simulink library "cvt_powertrain_lib"  (R2026a)
settings: Solver=VariableStepAuto
undefined symbols (not defined in the file or in its folder): fluids, HMPST
libraries: fl_lib x90, nesl_utility x31, cvt_components_lib x27, sdl_lib x24, SimscapeFluids_lib x11, simulink_extras x6, $bdroot x4, ee_lib x2, batteryecm_lib x1, simulink x1, engine_mgmt_lib x1, slpidlib x1
(part 3 of 4)

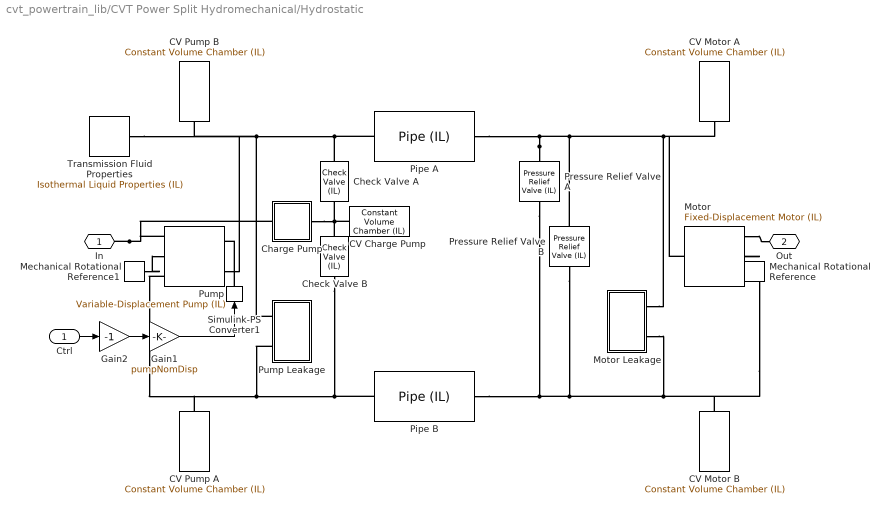
== system cvt_powertrain_lib/CVT Power Split Hydromechanical/Hydrostatic ==
  Ctrl : Inport
  CV Charge Pump : fl_lib/Isothermal Liquid/Elements/Constant Volume Chamber (IL)  volume=1e-4 m^3  p_I_specify=off  p_I_priority=High  p_I=0.101325 MPa  p_I_nominal_specify=off  p_I_nominal_value=1  p_I_nominal_unit=MPa
  CV Motor A : fl_lib/Isothermal Liquid/Elements/Constant Volume Chamber (IL)  volume=1e-4 m^3  p_I_specify=off  p_I_priority=High  p_I=0.101325 MPa  p_I_nominal_specify=off  p_I_nominal_value=1  p_I_nominal_unit=MPa
  CV Motor B : fl_lib/Isothermal Liquid/Elements/Constant Volume Chamber (IL)  volume=1e-4 m^3  p_I_specify=off  p_I_priority=High  p_I=0.101325 MPa  p_I_nominal_specify=off  p_I_nominal_value=1  p_I_nominal_unit=MPa
  CV Pump A : fl_lib/Isothermal Liquid/Elements/Constant Volume Chamber (IL)  volume=1e-4 m^3  p_I_specify=off  p_I_priority=High  p_I=0.101325 MPa  p_I_nominal_specify=off  p_I_nominal_value=1  p_I_nominal_unit=MPa
  CV Pump B : fl_lib/Isothermal Liquid/Elements/Constant Volume Chamber (IL)  volume=1e-4 m^3  p_I_specify=off  p_I_priority=High  p_I=0.101325 MPa  p_I_nominal_specify=off  p_I_nominal_value=1  p_I_nominal_unit=MPa
  Charge Pump : Subsystem  Tag=PublishSubsystem  mask{chgPumpNomDisp=chgPumpNomDisp, chgPumpNomSpd=chgPumpNomSpd, chgPumpNomPressGain=chgPumpNomPressGain, chgPumpNomVolEff=chgPumpNomVolEff, chgPumpNomMechEff=chgPumpNomMechEff, chgPumpChkvPdiff=chgPumpChkvPdiff, chgPumpChkvPrange=chgPumpChkvPrange, chgPumpChkvAmax=chgPumpChkvAmax, chgPumpChkvAleak=chgPumpChkvAleak}
      mask prompts: chgPumpNomDisp "Displacement (cm^3/rev)"; chgPumpNomSpd "Nominal Angular Velocity (rpm)"; chgPumpNomPressGain "Nominal pressure gain (MPa)"; chgPumpNomVolEff "Nominal Volumetric Efficiency (0-1)"; chgPumpNomMechEff "Nominal Mechanical Efficiency (0-1)"; chgPumpChkvPdiff "Set pressure differential (MPa)"; chgPumpChkvPrange "Pressure regulation range (MPa)"; chgPumpChkvAmax "Maximum opening area (m^2)"; chgPumpChkvAleak "Leakage area (m^2)"
      mask TypeOptions chgPumpNomDisp: Pump/displacement
      mask TypeOptions chgPumpNomSpd: Pump/omega_nominal
      mask TypeOptions chgPumpNomPressGain: Pump/p_nominal
      mask TypeOptions chgPumpNomVolEff: Pump/vol_eff_nominal
      mask TypeOptions chgPumpNomMechEff: Pump/mech_eff_nominal
      mask TypeOptions chgPumpChkvPdiff:
      | Pressure
      | Relief
      | Valve/p_set_differential
      mask TypeOptions chgPumpChkvPrange:
      | Pressure
      | Relief
      | Valve/p_range
      mask TypeOptions chgPumpChkvAmax:
      | Pressure
      | Relief
      | Valve/area_max
      mask TypeOptions chgPumpChkvAleak:
      | Pressure
      | Relief
      | Valve/area_leak
      mask DialogControl grp_chg_pump Prompt: Pump
      mask DialogControl grp_chg_pump_prv Prompt: Pressure Relief Valve
      mask Display:
      | % Circle
      | color('green')
      | plot(2*cos(linspace(0, 2*pi, 100)), 2*sin(linspace(0, 2*pi, 100)))
      | % Triangle
      | patch([1 0.4 0.4]*2, [0,-0.4,0.4]*2,[45 48 173]/255)
      | % Boundary
      | color('white')
      | plot(-2, -2)
      | plot(2, 2)
  Check Valve A : SimscapeFluids_lib/Isothermal Liquid/Valves & Orifices/Directional Control Valves/Check Valve (IL)  opening_spec=2*(fluids.isothermal_liquid.valves_orifices.enum.PressureOpeningSpec.Linear)-1  pressure_control_spec=fluids.isothermal_liquid.valves_orifices.enum.pressure_control_spec.dp  p_crack_differential=p_crack_differential MPa  p_crack_gauge=0.1 MPa  press_max_differential=press_max_differential MPa  press_max_gauge=0.2 MPa  area_max=chkv_area_max m^2  area_leak=chkv_area_leak m^2  p_diff_TLU=[0.01 : 0.01 : 0.1] MPa  valve_area_TLU=[1e-10, 1e-05, 2e-05, 3e-05, 4e-05, 5e-05, 6e-05, 7.5e-05, 8.5e-05, .0001] m^2  vol_flow_TLU=[.000358, .045, .11, .191, .284, .39, .505, .63, .764, .905] .* 1e-3 m^3/s  area=inf m^2  Cd=0.64  Re_c=150  smoothing_factor=0.01  pressure_recovery=simscape.enum.onoff.off  opening_dynamics=simscape.enum.onoff.off  tau=0.1 s
  Check Valve B : SimscapeFluids_lib/Isothermal Liquid/Valves & Orifices/Directional Control Valves/Check Valve (IL)  opening_spec=2*(fluids.isothermal_liquid.valves_orifices.enum.PressureOpeningSpec.Linear)-1  pressure_control_spec=fluids.isothermal_liquid.valves_orifices.enum.pressure_control_spec.dp  p_crack_differential=p_crack_differential MPa  p_crack_gauge=0.1 MPa  press_max_differential=press_max_differential MPa  press_max_gauge=0.2 MPa  area_max=chkv_area_max m^2  area_leak=chkv_area_leak m^2  p_diff_TLU=[0.01 : 0.01 : 0.1] MPa  valve_area_TLU=[1e-10, 1e-05, 2e-05, 3e-05, 4e-05, 5e-05, 6e-05, 7.5e-05, 8.5e-05, .0001] m^2  vol_flow_TLU=[.000358, .045, .11, .191, .284, .39, .505, .63, .764, .905] .* 1e-3 m^3/s  area=inf m^2  Cd=0.64  Re_c=150  smoothing_factor=0.01  pressure_recovery=simscape.enum.onoff.off  opening_dynamics=simscape.enum.onoff.off  tau=0.1 s
  Gain1 : Gain  Gain=pumpNomDisp
  Gain2 : Gain  Gain=-1
  Mechanical Rotational Reference : fl_lib/Mechanical/Rotational Elements/Mechanical Rotational Reference
  Mechanical Rotational Reference1 : fl_lib/Mechanical/Rotational Elements/Mechanical Rotational Reference
  Motor : SimscapeFluids_lib/Isothermal Liquid/Pumps & Motors/Fixed-Displacement Motor (IL)  leakage_friction_spec=fluids.isothermal_liquid.pumps_motors.enum.MotorLossSpec.Analytical  displacement=motorNomDisp cm^3/rev  omega_nominal=motorNomSpd rpm  p_nominal=motorNomPressDrop MPa  vol_eff_nominal=motorNomVolEff  mech_eff_nominal=motorNomMechEff  no_load_torque=0 N*m  p_diff_eff_TLU=[.1, 1, 2] MPa  omega_eff_TLU=[25, 50, 100, 200, 300, 400] rad/s  vol_eff_TLU=[.816, .908, .954, .977, .981, .984; .325, .663, .831, .916, .925, .946; .137, .568, .78, .892, .893, .91]  mech_eff_TLU=[.996, .996, .996, .996, .996, .996; .988, .989, .989, .989, .989, .99; .981, .981, .982, .982, .983, .984]  p_diff_loss_TLU=[.1, 1, 2] MPa  omega_loss_TLU=[25, 50, 100, 200, 300, 400] rad/s  vol_loss_TLU=[.023, .023, .023, .023, .0285, .032; .0844, .0842, .0845, .084, .1125, .108; .1079, .108, .11, .108, .1605, .18] * 1e-3 m^3/s  mech_loss_TLU=[.002, .002, .002, .002, .002, .002; .0607, .0556, .0556, .0556, .0556, .0505; .1937, .1937, .1833, .1833, .1729, .1626] N*m  q_shaft_TLU=[.125, .25, .5, 1, 1.5, 2] * 1e-3 m^3/s  p_diff_shaft_TLU=[.1, 1, 2] MPa  torque_shaft_TLU=[.47, 4.72, 9.35; .47, 4.7, 9.36; .47, 4.7, 9.4; .47, 4.7, 9.41; .47, 4.7, 9.46; .47, 4.68, 9.5] N*m  omega_shaft_TLU=[205, 80, 35; 455, 330, 285; 955, 831, 780; 1950, 1830, 1780; 2940, 2775, 2680; 3940, 3780, 3640] rpm  vol_eff_min=1e-3  vol_eff_max=1  mech_eff_min=1e-3  mech_eff_max=1  pressure_threshold=1e-3 MPa  omega_threshold=10 rad/s  supplied_range_check=simscape.enum.assert.action.none  motor_mode_check=simscape.enum.assert.action.none  pressure_check=simscape.enum.assert.action.none  p_min_valid=0.101325 MPa
  Motor Leakage : Subsystem  Tag=PublishSubsystem
  "Pipe A " : fl_lib/Isothermal Liquid/Elements/Pipe (IL)  length=pipeLen m  area=pipeAreaGeo m^2  Dh=pipeAreaHydr m  length_add=4 m  roughness=15e-6 m  Re_lam=2000  Re_tur=4000  shape_factor=64  dynamic_compressibility=simscape.enum.onoff.on  inertia=simscape.enum.onoff.off  p0=0.101325 MPa  mdot0=0 kg/s
  Pipe B : fl_lib/Isothermal Liquid/Elements/Pipe (IL)  length=pipeLen m  area=pipeAreaGeo m^2  Dh=pipeAreaHydr m  length_add=4 m  roughness=15e-6 m  Re_lam=2000  Re_tur=4000  shape_factor=64  dynamic_compressibility=simscape.enum.onoff.on  inertia=simscape.enum.onoff.off  p0=0.101325 MPa  mdot0=0 kg/s
  Pressure Relief Valve A : SimscapeFluids_lib/Isothermal Liquid/Valves & Orifices/Pressure Control Valves/Pressure Relief Valve (IL)  set_pressure_spec=foundation.enum.constant_controlled.constant  opening_spec=fluids.isothermal_liquid.valves_orifices.enum.opening_spec.linear  pressure_spec=fluids.isothermal_liquid.valves_orifices.enum.pressure_control_spec.dp  p_set_gauge=0.1 MPa  p_set_differential=p_set_differential MPa  p_range=p_range MPa  area_max=prv_area_max m^2  area_leak=prv_area_leak m^2  p_diff_TLU=[0.2 : 0.2 : 1.2] MPa  p_gauge_TLU=[0.2 : 0.2 : 1.2] MPa  valve_area_TLU=[1e-10, 2e-06, 4e-06, 6e-06, 8e-06, 1e-05] m^2  vol_flow_TLU=[1e-09, 3.6e-05, 8.9e-05, .00015, .00023, .00031] m^3/s  area=inf m^2  Cd=0.64  Re_c=150  smoothing_factor=0.01  pressure_recovery=simscape.enum.onoff.off  opening_dynamics=simscape.enum.onoff.off  tau=0.1 s
  Pressure Relief Valve B : SimscapeFluids_lib/Isothermal Liquid/Valves & Orifices/Pressure Control Valves/Pressure Relief Valve (IL)  set_pressure_spec=foundation.enum.constant_controlled.constant  opening_spec=fluids.isothermal_liquid.valves_orifices.enum.opening_spec.linear  pressure_spec=fluids.isothermal_liquid.valves_orifices.enum.pressure_control_spec.dp  p_set_gauge=0.1 MPa  p_set_differential=p_set_differential MPa  p_range=p_range MPa  area_max=prv_area_max m^2  area_leak=prv_area_leak m^2  p_diff_TLU=[0.2 : 0.2 : 1.2] MPa  p_gauge_TLU=[0.2 : 0.2 : 1.2] MPa  valve_area_TLU=[1e-10, 2e-06, 4e-06, 6e-06, 8e-06, 1e-05] m^2  vol_flow_TLU=[1e-09, 3.6e-05, 8.9e-05, .00015, .00023, .00031] m^3/s  area=inf m^2  Cd=0.64  Re_c=150  smoothing_factor=0.01  pressure_recovery=simscape.enum.onoff.off  opening_dynamics=simscape.enum.onoff.off  tau=0.1 s
  Pump : SimscapeFluids_lib/Isothermal Liquid/Pumps & Motors/Variable-Displacement Pump (IL)  leakage_friction_spec=fluids.isothermal_liquid.pumps_motors.enum.pump_motor_loss_spec.analytical  displacement_nominal=pumpNomDisp cm^3/rev  omega_nominal=pumpNomSpd rpm  p_nominal=pumpNomPressGain MPa  vol_eff_nominal=pumpNomVolEff  mech_eff_nominal=pumpNomMechEff  no_load_torque=0 N*m  p_diff_eff_TLU=[.1, 1, 2] MPa  omega_eff_TLU=[25, 50, 100, 200, 300, 400] rad/s  displacement_eff_TLU=[-30, -19, 19, 30] cm^3/rev  vol_eff_TLU=repmat([.816, .908, .954, .977, .981, .984; .325, .663, .831, .916, .925, .946; .137, .568, .78, .892, .893, .91], 1, 1, 4)  mech_eff_TLU=repmat([.996, .996, .996, .996, .996, .996; .988, .989, .989, .989, .989, .99; .981, .981, .982, .982, .983, .984], 1, 1, 4)  p_diff_loss_TLU=[.1, 1, 2] MPa  omega_loss_TLU=[25, 50, 100, 200, 300, 400] rad/s  displacement_loss_TLU=[-30, -19, 19, 30] cm^3/rev  vol_loss_TLU=repmat([.023, .023, .023, .023, .0285, .032; .0844, .0842, .0845, .084, .1125, .108; .1079, .108, .11, .108, .1605, .18] * 1e-3, 1, 1, 4) m^3/s  mech_loss_TLU=repmat([.002, .002, .002, .002, .002, .002; .0607, .0556, .0556, .0556, .0556, .0505; .1937, .1937, .1833, .1833, .1729, .1626], 1, 1, 4) N*m  vol_eff_min=1e-3  vol_eff_max=1  mech_eff_min=1e-3  mech_eff_max=1  pressure_threshold=1e-3 MPa  omega_threshold=10 rad/s  displacement_threshold=0.1 cm^3/rev  supplied_range_check=simscape.enum.assert.action.none  pump_mode_check=simscape.enum.assert.action.none  pressure_check=simscape.enum.assert.action.none  p_min_valid=0.101325 MPa
  Pump Leakage : Subsystem  Tag=PublishSubsystem
  Simulink-PS Converter1 : nesl_utility/Simulink-PS Converter  PhysicalDomain=network_engine_domain  SubClassName=ps_input  LeftPortType=input  RightPortType=output  PseudoPeriodic=off  Frequencies=[]  NoiseDistribution=none  NoiseParameters=[]  Unit=cm^3/rev  AffineConversion=off  FilteringAndDerivatives=provide  SimscapeFilterOrder=1  InputFilterTimeConstant=0.001  UdotUserProvided=0
  Transmission Fluid Properties : fl_lib/Isothermal Liquid/Utilities/Isothermal Liquid Properties (IL)  rho_L_atm=850 kg/m^3  bulk_modulus_model=foundation.enum.bulk_modulus_model.const  beta_gain=6  beta_L_atm=1.4 GPa  nu_atm=18.8 cSt  p_atm=0.101325 MPa  p_min=0.1 Pa  properties_range_check=simscape.enum.assert.action.error  air_fraction=0.005  polytropic_index=1.0  rho_g_atm=1.225 kg/m^3  air_dissolution_model=simscape.enum.onoff.off  p_crit=3 MPa
  In : PMIOPort  Side=Left
  Out : PMIOPort  Port=2  Side=Right
  wires:
  Ctrl/1 -> Gain2/1
  Gain1/1 -> Simulink-PS Converter1/1
  Gain2/1 -> Gain1/1
  connections:
  In/RConn1 -- Charge Pump/LConn1 -- Pump/RConn1
  Motor/RConn1 -- Out/RConn1
  Mechanical Rotational Reference1/LConn1 -- Pump/RConn2
  Pressure Relief Valve A/LConn1 -- Pressure Relief Valve B/RConn1 -- Motor Leakage/LConn1 -- CV Motor A/LConn1 -- Motor/LConn1 -- "Pipe A "/RConn1
  Motor/RConn2 -- Mechanical Rotational Reference/LConn1
  Check Valve B/LConn1 -- Check Valve A/LConn1 -- Charge Pump/RConn1 -- CV Charge Pump/LConn1
  Check Valve A/RConn1 -- Pump Leakage/LConn1 -- Transmission Fluid Properties/RConn1 -- CV Pump B/LConn1 -- Pump/LConn2 -- "Pipe A "/LConn1
  Check Valve B/RConn1 -- Pump Leakage/LConn2 -- CV Pump A/LConn1 -- Pump/RConn3 -- Pipe B/LConn1
  Pressure Relief Valve A/RConn1 -- Pressure Relief Valve B/LConn1 -- Motor Leakage/LConn2 -- CV Motor B/LConn1 -- Motor/RConn3 -- Pipe B/RConn1
  Simulink-PS Converter1/RConn1 -- Pump/LConn1

== system cvt_powertrain_lib/CVT Power Split Hydromechanical/Sensor P1s ==
  MRRef : fl_lib/Mechanical/Rotational Elements/Mechanical Rotational Reference
  Motion Sensor : fl_lib/Mechanical/Mechanical Sensors/Ideal Rotational Motion Sensor  reference=foundation.enum.MeasurementReference.difference  acceleration_port=false  velocity_port=true  position_port=false  wrap_angle=false  offset=0 rad
  PS-Simulink Converter : nesl_utility/PS-Simulink Converter  PhysicalDomain=network_engine_domain  SubClassName=ps_output  LeftPortType=input  RightPortType=output  PseudoPeriodic=off  Frequencies=[]  VectorFormat=inherit  Unit=rpm  AffineConversion=off
  R : PMIOPort  Side=Left
  w : Outport
  wires:
  PS-Simulink Converter/1 -> w/1
  connections:
  R/RConn1 -- Motion Sensor/LConn1
  MRRef/LConn1 -- Motion Sensor/RConn1
  PS-Simulink Converter/LConn1 -- Motion Sensor/RConn2

== system cvt_powertrain_lib/CVT Power Split Hydromechanical/Sensor wG2 ==
  MRRef : fl_lib/Mechanical/Rotational Elements/Mechanical Rotational Reference
  Motion Sensor : fl_lib/Mechanical/Mechanical Sensors/Ideal Rotational Motion Sensor  reference=foundation.enum.MeasurementReference.difference  acceleration_port=false  velocity_port=true  position_port=false  wrap_angle=false  offset=0 rad
  PS-Simulink Converter : nesl_utility/PS-Simulink Converter  PhysicalDomain=network_engine_domain  SubClassName=ps_output  LeftPortType=input  RightPortType=output  PseudoPeriodic=off  Frequencies=[]  VectorFormat=inherit  Unit=rpm  AffineConversion=off
  R : PMIOPort  Side=Left
  w : Outport
  wires:
  PS-Simulink Converter/1 -> w/1
  connections:
  R/RConn1 -- Motion Sensor/LConn1
  MRRef/LConn1 -- Motion Sensor/RConn1
  PS-Simulink Converter/LConn1 -- Motion Sensor/RConn2

== system cvt_powertrain_lib/CVT Power Split Hydromechanical/Sensor wG3 ==
  MRRef : fl_lib/Mechanical/Rotational Elements/Mechanical Rotational Reference
  Motion Sensor : fl_lib/Mechanical/Mechanical Sensors/Ideal Rotational Motion Sensor  reference=foundation.enum.MeasurementReference.difference  acceleration_port=false  velocity_port=true  position_port=false  wrap_angle=false  offset=0 rad
  PS-Simulink Converter : nesl_utility/PS-Simulink Converter  PhysicalDomain=network_engine_domain  SubClassName=ps_output  LeftPortType=input  RightPortType=output  PseudoPeriodic=off  Frequencies=[]  VectorFormat=inherit  Unit=rpm  AffineConversion=off
  R : PMIOPort  Side=Left
  w : Outport
  wires:
  PS-Simulink Converter/1 -> w/1
  connections:
  PS-Simulink Converter/LConn1 -- Motion Sensor/RConn2
  MRRef/LConn1 -- Motion Sensor/RConn1
  R/RConn1 -- Motion Sensor/LConn1

== system cvt_powertrain_lib/CVT Power Split Hydromechanical/Sensor wG4 ==
  MRRef : fl_lib/Mechanical/Rotational Elements/Mechanical Rotational Reference
  Motion Sensor : fl_lib/Mechanical/Mechanical Sensors/Ideal Rotational Motion Sensor  reference=foundation.enum.MeasurementReference.difference  acceleration_port=false  velocity_port=true  position_port=false  wrap_angle=false  offset=0 rad
  PS-Simulink Converter : nesl_utility/PS-Simulink Converter  PhysicalDomain=network_engine_domain  SubClassName=ps_output  LeftPortType=input  RightPortType=output  PseudoPeriodic=off  Frequencies=[]  VectorFormat=inherit  Unit=rpm  AffineConversion=off
  R : PMIOPort  Side=Left
  w : Outport
  wires:
  PS-Simulink Converter/1 -> w/1
  connections:
  PS-Simulink Converter/LConn1 -- Motion Sensor/RConn2
  MRRef/LConn1 -- Motion Sensor/RConn1
  R/RConn1 -- Motion Sensor/LConn1

== system cvt_powertrain_lib/CVT Power Split Hydromechanical/Sensor wIn ==
  MRRef : fl_lib/Mechanical/Rotational Elements/Mechanical Rotational Reference
  Motion Sensor : fl_lib/Mechanical/Mechanical Sensors/Ideal Rotational Motion Sensor  reference=foundation.enum.MeasurementReference.difference  acceleration_port=false  velocity_port=true  position_port=false  wrap_angle=false  offset=0 rad
  PS-Simulink Converter : nesl_utility/PS-Simulink Converter  PhysicalDomain=network_engine_domain  SubClassName=ps_output  LeftPortType=input  RightPortType=output  PseudoPeriodic=off  Frequencies=[]  VectorFormat=inherit  Unit=rpm  AffineConversion=off
  R : PMIOPort  Side=Left
  w : Outport
  wires:
  PS-Simulink Converter/1 -> w/1
  connections:
  PS-Simulink Converter/LConn1 -- Motion Sensor/RConn2
  MRRef/LConn1 -- Motion Sensor/RConn1
  R/RConn1 -- Motion Sensor/LConn1

== system cvt_powertrain_lib/CVT Power Split Hydromechanical/Sensor wOut ==
  MRRef : fl_lib/Mechanical/Rotational Elements/Mechanical Rotational Reference
  Motion Sensor : fl_lib/Mechanical/Mechanical Sensors/Ideal Rotational Motion Sensor  reference=foundation.enum.MeasurementReference.difference  acceleration_port=false  velocity_port=true  position_port=false  wrap_angle=false  offset=0 rad
  PS-Simulink Converter : nesl_utility/PS-Simulink Converter  PhysicalDomain=network_engine_domain  SubClassName=ps_output  LeftPortType=input  RightPortType=output  PseudoPeriodic=off  Frequencies=[]  VectorFormat=inherit  Unit=rpm  AffineConversion=off
  R : PMIOPort  Side=Left
  w : Outport
  wires:
  PS-Simulink Converter/1 -> w/1
  connections:
  R/RConn1 -- Motion Sensor/LConn1
  MRRef/LConn1 -- Motion Sensor/RConn1
  PS-Simulink Converter/LConn1 -- Motion Sensor/RConn2

== system cvt_powertrain_lib/CVT Power Split Hydromechanical/Sensor wP1c ==
  MRRef : fl_lib/Mechanical/Rotational Elements/Mechanical Rotational Reference
  Motion Sensor : fl_lib/Mechanical/Mechanical Sensors/Ideal Rotational Motion Sensor  reference=foundation.enum.MeasurementReference.difference  acceleration_port=false  velocity_port=true  position_port=false  wrap_angle=false  offset=0 rad
  PS-Simulink Converter : nesl_utility/PS-Simulink Converter  PhysicalDomain=network_engine_domain  SubClassName=ps_output  LeftPortType=input  RightPortType=output  PseudoPeriodic=off  Frequencies=[]  VectorFormat=inherit  Unit=rpm  AffineConversion=off
  R : PMIOPort  Side=Left
  w : Outport
  wires:
  PS-Simulink Converter/1 -> w/1
  connections:
  R/RConn1 -- Motion Sensor/LConn1
  MRRef/LConn1 -- Motion Sensor/RConn1
  PS-Simulink Converter/LConn1 -- Motion Sensor/RConn2

== system cvt_powertrain_lib/CVT Power Split Hydromechanical/Sensor wP2s ==
  MRRef : fl_lib/Mechanical/Rotational Elements/Mechanical Rotational Reference
  Motion Sensor : fl_lib/Mechanical/Mechanical Sensors/Ideal Rotational Motion Sensor  reference=foundation.enum.MeasurementReference.difference  acceleration_port=false  velocity_port=true  position_port=false  wrap_angle=false  offset=0 rad
  PS-Simulink Converter : nesl_utility/PS-Simulink Converter  PhysicalDomain=network_engine_domain  SubClassName=ps_output  LeftPortType=input  RightPortType=output  PseudoPeriodic=off  Frequencies=[]  VectorFormat=inherit  Unit=rpm  AffineConversion=off
  R : PMIOPort  Side=Left
  w : Outport
  wires:
  PS-Simulink Converter/1 -> w/1
  connections:
  PS-Simulink Converter/LConn1 -- Motion Sensor/RConn2
  MRRef/LConn1 -- Motion Sensor/RConn1
  R/RConn1 -- Motion Sensor/LConn1

== system cvt_powertrain_lib/CVT Power Split Hydromechanical/Sensor wP3r ==
  MRRef : fl_lib/Mechanical/Rotational Elements/Mechanical Rotational Reference
  Motion Sensor : fl_lib/Mechanical/Mechanical Sensors/Ideal Rotational Motion Sensor  reference=foundation.enum.MeasurementReference.difference  acceleration_port=false  velocity_port=true  position_port=false  wrap_angle=false  offset=0 rad
  PS-Simulink Converter : nesl_utility/PS-Simulink Converter  PhysicalDomain=network_engine_domain  SubClassName=ps_output  LeftPortType=input  RightPortType=output  PseudoPeriodic=off  Frequencies=[]  VectorFormat=inherit  Unit=rpm  AffineConversion=off
  R : PMIOPort  Side=Left
  w : Outport
  wires:
  PS-Simulink Converter/1 -> w/1
  connections:
  PS-Simulink Converter/LConn1 -- Motion Sensor/RConn2
  MRRef/LConn1 -- Motion Sensor/RConn1
  R/RConn1 -- Motion Sensor/LConn1

== system cvt_powertrain_lib/CVT Power Split Hydromechanical/Sensor wP4c ==
  MRRef : fl_lib/Mechanical/Rotational Elements/Mechanical Rotational Reference
  Motion Sensor : fl_lib/Mechanical/Mechanical Sensors/Ideal Rotational Motion Sensor  reference=foundation.enum.MeasurementReference.difference  acceleration_port=false  velocity_port=true  position_port=false  wrap_angle=false  offset=0 rad
  PS-Simulink Converter : nesl_utility/PS-Simulink Converter  PhysicalDomain=network_engine_domain  SubClassName=ps_output  LeftPortType=input  RightPortType=output  PseudoPeriodic=off  Frequencies=[]  VectorFormat=inherit  Unit=rpm  AffineConversion=off
  R : PMIOPort  Side=Left
  w : Outport
  wires:
  PS-Simulink Converter/1 -> w/1
  connections:
  PS-Simulink Converter/LConn1 -- Motion Sensor/RConn2
  MRRef/LConn1 -- Motion Sensor/RConn1
  R/RConn1 -- Motion Sensor/LConn1

== system cvt_powertrain_lib/CVT Power Split Hydromechanical/Sensor wP4r ==
  MRRef : fl_lib/Mechanical/Rotational Elements/Mechanical Rotational Reference
  Motion Sensor : fl_lib/Mechanical/Mechanical Sensors/Ideal Rotational Motion Sensor  reference=foundation.enum.MeasurementReference.difference  acceleration_port=false  velocity_port=true  position_port=false  wrap_angle=false  offset=0 rad
  PS-Simulink Converter : nesl_utility/PS-Simulink Converter  PhysicalDomain=network_engine_domain  SubClassName=ps_output  LeftPortType=input  RightPortType=output  PseudoPeriodic=off  Frequencies=[]  VectorFormat=inherit  Unit=rpm  AffineConversion=off
  R : PMIOPort  Side=Left
  w : Outport
  wires:
  PS-Simulink Converter/1 -> w/1
  connections:
  R/RConn1 -- Motion Sensor/LConn1
  MRRef/LConn1 -- Motion Sensor/RConn1
  PS-Simulink Converter/LConn1 -- Motion Sensor/RConn2

== system cvt_powertrain_lib/CVT Power Split Hydromechanical/Sensor wP4s ==
  MRRef : fl_lib/Mechanical/Rotational Elements/Mechanical Rotational Reference
  Motion Sensor : fl_lib/Mechanical/Mechanical Sensors/Ideal Rotational Motion Sensor  reference=foundation.enum.MeasurementReference.difference  acceleration_port=false  velocity_port=true  position_port=false  wrap_angle=false  offset=0 rad
  PS-Simulink Converter : nesl_utility/PS-Simulink Converter  PhysicalDomain=network_engine_domain  SubClassName=ps_output  LeftPortType=input  RightPortType=output  PseudoPeriodic=off  Frequencies=[]  VectorFormat=inherit  Unit=rpm  AffineConversion=off
  R : PMIOPort  Side=Left
  w : Outport
  wires:
  PS-Simulink Converter/1 -> w/1
  connections:
  PS-Simulink Converter/LConn1 -- Motion Sensor/RConn2
  MRRef/LConn1 -- Motion Sensor/RConn1
  R/RConn1 -- Motion Sensor/LConn1

== system cvt_powertrain_lib/Controller/CVT Ratio Ctrl ==
  Ratio (-) : Inport
  CmdVehSpdDir : Inport  Port=2
  HRBCtrl (-) : Inport  Port=3
  MBCtrl (-) : Inport  Port=4
  Bus Creator : BusCreator  Inputs=12
  Clutch Truth Table : Stateflow chart  TreatAsAtomicUnit=on
  Filter : StateSpace  A=-200  C=200  D=0  InitialCondition=HMPST.Ctrl.Swash.XY_A(1,1)/200
  Range Calculation : Subsystem  mask{XY_I=HMPST.Ctrl.Swash.XY_I}
      mask prompts: XY_I "Range Separation Points"
  Saturation : Saturate  UpperLimit=HMPST.DesignReq.MaxCVTOutputSpeed/HMPST.Eng.wTarget  LowerLimit=0  ZeroCross=off
  Swash Ctrl : Lookup_n-D  NumberOfTableDimensions=1  BreakpointsForDimension1=HMPST.Ctrl.Swash.XY_A(:,2)  BeginIndexSearchUsingPreviousIndexResult=on  Table=HMPST.Ctrl.Swash.XY_A(:,1)  InternalRulePriority=Speed  RndMeth=Simplest
  Transfer Fcn : TransferFcn  Denominator=[0.1 1]
  CVT Ctrl : Outport
  wires:
  Ratio (-)/1 -> [ratio], Transfer Fcn/1
  Clutch Truth Table/1(K1Actv) -> Bus Creator/1  "K1"
  Clutch Truth Table/2(K2Actv) -> Bus Creator/2  "K2"
  Clutch Truth Table/3(K3Actv) -> Bus Creator/3  "K3"
  Clutch Truth Table/4(K4Actv) -> Bus Creator/4  "K4"
  Clutch Truth Table/5(KbActv) -> Bus Creator/5  "Kb"
  Clutch Truth Table/6(KvActv) -> Bus Creator/6  "Kv"
  Clutch Truth Table/7(KrActv) -> Bus Creator/7  "Kr"
  Bus Creator/1 -> CVT Ctrl/1  "Ctrl"
  Range Calculation/1(Range (-)) -> Clutch Truth Table/1(Range)
  Saturation/1 -> Swash Ctrl/1, Range Calculation/1(Ratio (-))
  Transfer Fcn/1 -> Saturation/1
  Filter/1 -> Bus Creator/12  "SwashCtrl"
  Swash Ctrl/1 -> Filter/1  "SwashCtrl"
  HRBCtrl (-)/1 -> Bus Creator/8  "HRBCtrl"
  MBCtrl (-)/1 -> Bus Creator/9  "MBCtrl"
  CmdVehSpdDir/1 -> Bus Creator/11, Clutch Truth Table/2(CmdVehSpdDir)  "CmdVehSpdDir"
  [ratio] -> Bus Creator/10  "ratio"

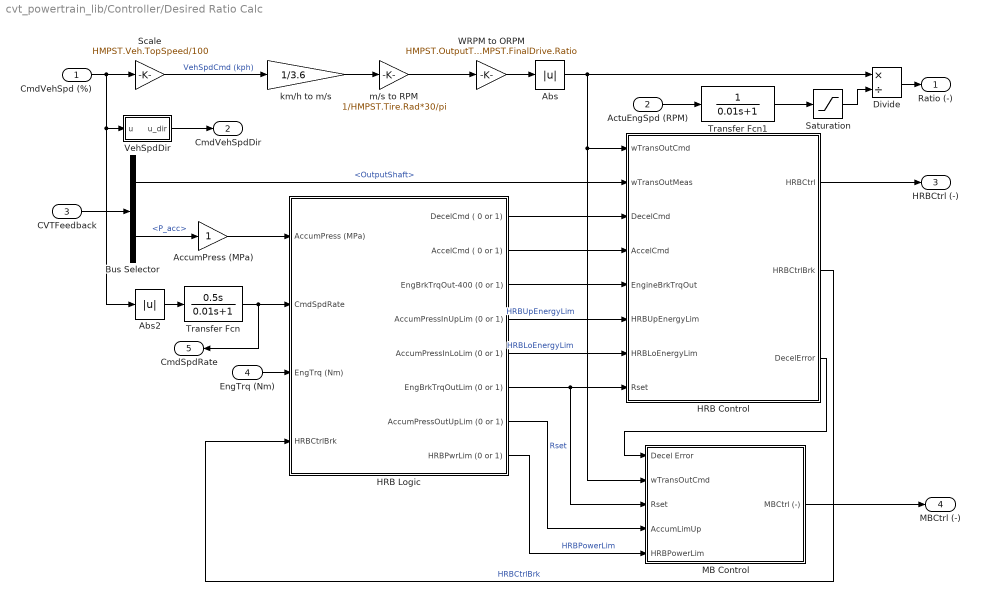
== system cvt_powertrain_lib/Controller/Desired Ratio Calc ==
  CmdVehSpd (%) : Inport  SampleTime=HMPST.Simu.TimeStep
  ActuEngSpd (RPM) : Inport  Port=2
  CVTFeedback : Inport  Port=3
  EngTrq (Nm) : Inport  Port=4
  Abs : Abs  ZeroCross=off  SaturateOnIntegerOverflow=off
  Abs2 : Abs  ZeroCross=off  SaturateOnIntegerOverflow=off
  AccumPress (MPa) : Gain
  Bus Selector : BusSelector  OutputSignals=OutputShaft,P_acc
  Divide : Product  Inputs=*/
  HRB Control : Subsystem
  HRB Logic : Subsystem
  MB Control : Subsystem
  Saturation : Saturate  UpperLimit=2500  LowerLimit=0.5
  Scale : Gain  Gain=HMPST.Veh.TopSpeed/100
  Transfer Fcn : TransferFcn  Numerator=[0.5 0]  Denominator=[0.01 1]
  Transfer Fcn1 : TransferFcn  Denominator=[0.01 1]
  VehSpdDir : Subsystem
  WRPM to ORPM : Gain  Gain=HMPST.OutputTransferGearPair.Ratio*HMPST.Differential.Ratio*HMPST.FinalDrive.Ratio
  km/h to m/s : Gain  Gain=1/3.6
  m/s to RPM : Gain  Gain=1/HMPST.Tire.Rad*30/pi
  Ratio (-) : Outport
  CmdVehSpdDir : Outport  Port=2
  HRBCtrl (-) : Outport  Port=3
  MBCtrl (-) : Outport  Port=4
  CmdSpdRate : Outport  Port=5
  wires:
  HRB Logic/8(HRBPwrLim (0 or 1)) -> MB Control/5(HRBPowerLim)  "HRBPowerLim"
  HRB Logic/7(AccumPressOutUpLim (0 or 1)) -> MB Control/4(AccumLimUp)
  HRB Control/3(DecelError) -> MB Control/1(Decel Error)
  HRB Control/1(HRBCtrl) -> HRBCtrl (-)/1
  HRB Logic/3(EngBrkTrqOut-400 (0 or 1)) -> HRB Control/5(EngineBrkTrqOut)
  HRB Logic/2(AccelCmd ( 0 or 1)) -> HRB Control/4(AccelCmd)
  HRB Logic/5(AccumPressInLoLim (0 or 1)) -> HRB Control/7(HRBLoEnergyLim)  "HRBLoEnergyLim"
  HRB Logic/4(AccumPressInUpLim (0 or 1)) -> HRB Control/6(HRBUpEnergyLim)  "HRBUpEnergyLim"
  HRB Logic/1(DecelCmd ( 0 or 1)) -> HRB Control/3(DecelCmd)
  Divide/1 -> Ratio (-)/1
  ActuEngSpd (RPM)/1 -> Transfer Fcn1/1
  m/s to RPM/1 -> WRPM to ORPM/1
  km/h to m/s/1 -> m/s to RPM/1
  WRPM to ORPM/1 -> Abs/1
  CmdVehSpd (%)/1 -> Abs2/1, VehSpdDir/1(u), Scale/1
  Saturation/1 -> Divide/2
  Transfer Fcn1/1 -> Saturation/1
  Bus Selector/1 -> HRB Control/2(wTransOutMeas)  "<OutputShaft>"
  Transfer Fcn/1 -> HRB Logic/2(CmdSpdRate), CmdSpdRate/1
  CVTFeedback/1 -> Bus Selector/1
  HRB Logic/6(EngBrkTrqOutLim (0 or 1)) -> MB Control/3(Rset), HRB Control/8(Rset)  "Rset"
  Bus Selector/2 -> AccumPress (MPa)/1  "<P_acc>"
  EngTrq (Nm)/1 -> HRB Logic/3(EngTrq (Nm))
  AccumPress (MPa)/1 -> HRB Logic/1(AccumPress (MPa))
  VehSpdDir/1(u_dir) -> CmdVehSpdDir/1
  Scale/1 -> km/h to m/s/1  "VehSpdCmd (kph)"
  Abs2/1 -> Transfer Fcn/1
  Abs/1 -> Divide/1, MB Control/2(wTransOutCmd), HRB Control/1(wTransOutCmd)
  MB Control/1(MBCtrl (-)) -> MBCtrl (-)/1
  HRB Control/2(HRBCtrlBrk) -> HRB Logic/4(HRBCtrlBrk)  "HRBCtrlBrk"

== system cvt_powertrain_lib/Driveline/Compliance FL ==
  Damper : fl_lib/Mechanical/Rotational Elements/Rotational Damper  D=HMPST.DriveshaftF.D N*m*s/rad  w_specify=off  w_priority=None  w=0 rad/s  w_nominal_specify=off  w_nominal_value=1  w_nominal_unit=rad/s  t_specify=off  t_priority=None  t=0 N*m  t_nominal_specify=off  t_nominal_value=1  t_nominal_unit=N*m
  Spring : fl_lib/Mechanical/Rotational Elements/Rotational Spring  spr_rate=HMPST.DriveshaftF.K N*m/rad  w_specify=off  w_priority=None  w=0 rad/s  w_nominal_specify=off  w_nominal_value=1  w_nominal_unit=rad/s  t_specify=off  t_priority=None  t=0 N*m  t_nominal_specify=off  t_nominal_value=1  t_nominal_unit=N*m  phi_specify=off  phi_priority=High  phi=0 rad  phi_nominal_specify=off  phi_nominal_value=1  phi_nominal_unit=rad
  R : PMIOPort  Side=Right
  C : PMIOPort  Port=2  Side=Left
  connections:
  Damper/LConn1 -- Spring/LConn1 -- R/RConn1
  Damper/RConn1 -- Spring/RConn1 -- C/RConn1

== system cvt_powertrain_lib/Driveline/Compliance FR ==
  Damper : fl_lib/Mechanical/Rotational Elements/Rotational Damper  D=HMPST.DriveshaftF.D N*m*s/rad  w_specify=off  w_priority=None  w=0 rad/s  w_nominal_specify=off  w_nominal_value=1  w_nominal_unit=rad/s  t_specify=off  t_priority=None  t=0 N*m  t_nominal_specify=off  t_nominal_value=1  t_nominal_unit=N*m
  Spring : fl_lib/Mechanical/Rotational Elements/Rotational Spring  spr_rate=HMPST.DriveshaftF.K N*m/rad  w_specify=off  w_priority=None  w=0 rad/s  w_nominal_specify=off  w_nominal_value=1  w_nominal_unit=rad/s  t_specify=off  t_priority=None  t=0 N*m  t_nominal_specify=off  t_nominal_value=1  t_nominal_unit=N*m  phi_specify=off  phi_priority=High  phi=0 rad  phi_nominal_specify=off  phi_nominal_value=1  phi_nominal_unit=rad
  R : PMIOPort  Side=Right
  C : PMIOPort  Port=2  Side=Left
  connections:
  C/RConn1 -- Damper/RConn1 -- Spring/RConn1
  R/RConn1 -- Spring/LConn1 -- Damper/LConn1

== system cvt_powertrain_lib/Driveline/Compliance RL ==
  Damper : fl_lib/Mechanical/Rotational Elements/Rotational Damper  D=HMPST.DriveshaftF.D N*m*s/rad  w_specify=off  w_priority=None  w=0 rad/s  w_nominal_specify=off  w_nominal_value=1  w_nominal_unit=rad/s  t_specify=off  t_priority=None  t=0 N*m  t_nominal_specify=off  t_nominal_value=1  t_nominal_unit=N*m
  Spring : fl_lib/Mechanical/Rotational Elements/Rotational Spring  spr_rate=HMPST.DriveshaftF.K N*m/rad  w_specify=off  w_priority=None  w=0 rad/s  w_nominal_specify=off  w_nominal_value=1  w_nominal_unit=rad/s  t_specify=off  t_priority=None  t=0 N*m  t_nominal_specify=off  t_nominal_value=1  t_nominal_unit=N*m  phi_specify=off  phi_priority=High  phi=0 rad  phi_nominal_specify=off  phi_nominal_value=1  phi_nominal_unit=rad
  R : PMIOPort  Side=Right
  C : PMIOPort  Port=2  Side=Left
  connections:
  C/RConn1 -- Damper/RConn1 -- Spring/RConn1
  R/RConn1 -- Spring/LConn1 -- Damper/LConn1

== system cvt_powertrain_lib/Driveline/Compliance RR ==
  Damper : fl_lib/Mechanical/Rotational Elements/Rotational Damper  D=HMPST.DriveshaftF.D N*m*s/rad  w_specify=off  w_priority=None  w=0 rad/s  w_nominal_specify=off  w_nominal_value=1  w_nominal_unit=rad/s  t_specify=off  t_priority=None  t=0 N*m  t_nominal_specify=off  t_nominal_value=1  t_nominal_unit=N*m
  Spring : fl_lib/Mechanical/Rotational Elements/Rotational Spring  spr_rate=HMPST.DriveshaftF.K N*m/rad  w_specify=off  w_priority=None  w=0 rad/s  w_nominal_specify=off  w_nominal_value=1  w_nominal_unit=rad/s  t_specify=off  t_priority=None  t=0 N*m  t_nominal_specify=off  t_nominal_value=1  t_nominal_unit=N*m  phi_specify=off  phi_priority=High  phi=0 rad  phi_nominal_specify=off  phi_nominal_value=1  phi_nominal_unit=rad
  R : PMIOPort  Side=Right
  C : PMIOPort  Port=2  Side=Left
  connections:
  C/RConn1 -- Damper/RConn1 -- Spring/RConn1
  R/RConn1 -- Spring/LConn1 -- Damper/LConn1

== system cvt_powertrain_lib/Engine Droop/Speed Sensor ==
  MRRef : fl_lib/Mechanical/Rotational Elements/Mechanical Rotational Reference
  Motion Sensor : fl_lib/Mechanical/Mechanical Sensors/Ideal Rotational Motion Sensor  reference=foundation.enum.MeasurementReference.difference  acceleration_port=false  velocity_port=true  position_port=false  wrap_angle=false  offset=0 rad
  Press A3 : nesl_utility/PS-Simulink Converter  PhysicalDomain=network_engine_domain  SubClassName=ps_output  LeftPortType=input  RightPortType=output  PseudoPeriodic=off  Frequencies=[]  VectorFormat=1-D array  Unit=rpm  AffineConversion=off
  Transfer Fcn : TransferFcn  Denominator=[0.1 1]
  R : PMIOPort  Side=Left
  rpm : Outport
  wires:
  Transfer Fcn/1 -> rpm/1
  Press A3/1 -> Transfer Fcn/1
  connections:
  R/RConn1 -- Motion Sensor/LConn1
  MRRef/LConn1 -- Motion Sensor/RConn1
  Motion Sensor/RConn2 -- Press A3/LConn1

== system cvt_powertrain_lib/Engine Droop/Torque Sensor ==
  PS-Simulink Converter : nesl_utility/PS-Simulink Converter  PhysicalDomain=network_engine_domain  SubClassName=ps_output  LeftPortType=input  RightPortType=output  PseudoPeriodic=off  Frequencies=[]  VectorFormat=inherit  Unit=inherit  AffineConversion=off
  Torque Sensor : fl_lib/Mechanical/Mechanical Sensors/Ideal Torque Sensor
  R : PMIOPort  Side=Left
  C : PMIOPort  Port=2  Side=Right
  m : Outport
  wires:
  PS-Simulink Converter/1 -> m/1
  connections:
  PS-Simulink Converter/LConn1 -- Torque Sensor/RConn2
  Torque Sensor/LConn1 -- R/RConn1
  C/RConn1 -- Torque Sensor/RConn1

== system cvt_powertrain_lib/Engine Generic/Speed Sensor ==
  Ideal Rotational Motion Sensor1 : fl_lib/Mechanical/Mechanical Sensors/Ideal Rotational Motion Sensor  reference=foundation.enum.MeasurementReference.difference  acceleration_port=false  velocity_port=true  position_port=false  wrap_angle=false  offset=0 rad
  Mechanical Rotational Reference1 : fl_lib/Mechanical/Rotational Elements/Mechanical Rotational Reference
  Press A3 : nesl_utility/PS-Simulink Converter  PhysicalDomain=network_engine_domain  SubClassName=ps_output  LeftPortType=input  RightPortType=output  PseudoPeriodic=off  Frequencies=[]  VectorFormat=1-D array  Unit=rpm  AffineConversion=off
  Transfer Fcn : TransferFcn  Denominator=[0.1 1]
  R : PMIOPort  Side=Left
  w (rpm) : Outport
  wires:
  Transfer Fcn/1 -> w (rpm)/1
  Press A3/1 -> Transfer Fcn/1
  connections:
  R/RConn1 -- Ideal Rotational Motion Sensor1/LConn1
  Mechanical Rotational Reference1/LConn1 -- Ideal Rotational Motion Sensor1/RConn1
  Ideal Rotational Motion Sensor1/RConn2 -- Press A3/LConn1

== system cvt_powertrain_lib/Engine Generic/Subsystem ==
  Ideal Torque Sensor : fl_lib/Mechanical/Mechanical Sensors/Ideal Torque Sensor
  PS-Simulink Converter : nesl_utility/PS-Simulink Converter  PhysicalDomain=network_engine_domain  SubClassName=ps_output  LeftPortType=input  RightPortType=output  PseudoPeriodic=off  Frequencies=[]  VectorFormat=inherit  Unit=inherit  AffineConversion=off
  R : PMIOPort  Side=Left
  C : PMIOPort  Port=2  Side=Right
  m : Outport
  wires:
  PS-Simulink Converter/1 -> m/1
  connections:
  PS-Simulink Converter/LConn1 -- Ideal Torque Sensor/RConn2
  Ideal Torque Sensor/LConn1 -- R/RConn1
  C/RConn1 -- Ideal Torque Sensor/RConn1

== system cvt_powertrain_lib/CVT Electrical/Control/Control ==
  wCmd : Inport
  wMeas : Inport  Port=2
  Integrator : Integrator
  Ki : Gain  Gain=HMPST.eCVT.Control.Ki
  Kp : Gain  Gain=HMPST.eCVT.Control.Kp
  Sum : Sum  Inputs=+-|
  Sum1 : Sum  Inputs=++|
  Transfer Fcn (with initial states) : simulink_extras/Additional Linear/Transfer Fcn (with initial states)  N=[1]  D="[HMPST.eCVT.Control.tFilt  1]"  X0=0
  Trq : Outport
  wires:
  Sum/1 -> Transfer Fcn (with initial states)/1
  Sum1/1 -> Trq/1
  Kp/1 -> Sum1/2
  Ki/1 -> Integrator/1
  Integrator/1 -> Sum1/1
  Transfer Fcn (with initial states)/1 -> Ki/1, Kp/1
  wMeas/1 -> Sum/2
  wCmd/1 -> Sum/1

== system cvt_powertrain_lib/CVT Power Split Hydromechanical/HRB/Subsystem ==
  Hydraulic Pressure Sensor : fl_lib/Isothermal Liquid/Sensors/Pressure Sensor (IL)  pressure_measure=foundation.enum.pressure_measure.difference
      settings: LibrarySourceBlock=|
      | fl_lib/Hydraulic/Hydraulic Sensors/Hydraulic Pressure
      | Sensor
  Hydraulic Reference1 : fl_lib/Isothermal Liquid/Elements/Reservoir (IL)  pressure_input=false  pressure_spec=foundation.enum.pressure_spec.atmospheric  reservoir_pressure=0.101325 MPa
      settings: LibrarySourceBlock=fl_lib/Hydraulic/Hydraulic Elements/Hydraulic Reference
  PS-Simulink Converter : nesl_utility/PS-Simulink Converter  PhysicalDomain=network_engine_domain  SubClassName=ps_output  LeftPortType=input  RightPortType=output  PseudoPeriodic=off  Frequencies=[]  VectorFormat=1-D array  Unit=MPa  AffineConversion=off
  A : PMIOPort  Side=Left
  p : Outport
  wires:
  PS-Simulink Converter/1 -> p/1
  connections:
  Hydraulic Pressure Sensor/RConn1 -- Hydraulic Reference1/LConn1
  A/RConn1 -- Hydraulic Pressure Sensor/LConn1
  Hydraulic Pressure Sensor/RConn2 -- PS-Simulink Converter/LConn1

== system cvt_powertrain_lib/CVT Power Split Hydromechanical/Hydrostatic/Charge Pump ==
  Mechanical Rotational Reference : fl_lib/Mechanical/Rotational Elements/Mechanical Rotational Reference
  Pressure Relief Valve : SimscapeFluids_lib/Isothermal Liquid/Valves & Orifices/Pressure Control Valves/Pressure Relief Valve (IL)  set_pressure_spec=foundation.enum.constant_controlled.constant  opening_spec=fluids.isothermal_liquid.valves_orifices.enum.opening_spec.linear  pressure_spec=fluids.isothermal_liquid.valves_orifices.enum.pressure_control_spec.dp  p_set_gauge=0.1 MPa  p_set_differential=chgPumpChkvPdiff MPa  p_range=chgPumpChkvPrange MPa  area_max=chgPumpChkvAmax m^2  area_leak=chgPumpChkvAleak m^2  p_diff_TLU=[0.2 : 0.2 : 1.2] MPa  p_gauge_TLU=[0.2 : 0.2 : 1.2] MPa  valve_area_TLU=[1e-10, 2e-06, 4e-06, 6e-06, 8e-06, 1e-05] m^2  vol_flow_TLU=[1e-09, 3.6e-05, 8.9e-05, .00015, .00023, .00031] m^3/s  area=inf m^2  Cd=0.64  Re_c=150  smoothing_factor=0.01  pressure_recovery=simscape.enum.onoff.off  opening_dynamics=simscape.enum.onoff.off  tau=0.1 s
  Pump : SimscapeFluids_lib/Isothermal Liquid/Pumps & Motors/Fixed-Displacement Pump (IL)  leakage_friction_spec=fluids.isothermal_liquid.pumps_motors.enum.pump_motor_loss_spec.analytical  displacement=chgPumpNomDisp cm^3/rev  omega_nominal=chgPumpNomSpd rpm  p_nominal=chgPumpNomPressGain MPa  vol_eff_nominal=chgPumpNomVolEff  mech_eff_nominal=chgPumpNomMechEff  no_load_torque=0 N*m  p_diff_eff_TLU=[.1, 1, 2] MPa  omega_eff_TLU=[25, 50, 100, 200, 300, 400] rad/s  vol_eff_TLU=[.816, .908, .954, .977, .981, .984; .325, .663, .831, .916, .925, .946; .137, .568, .78, .892, .893, .91]  mech_eff_TLU=[.996, .996, .996, .996, .996, .996; .988, .989, .989, .989, .989, .99; .981, .981, .982, .982, .983, .984]  p_diff_loss_TLU=[.1, 1, 2] MPa  omega_loss_TLU=[25, 50, 100, 200, 300, 400] rad/s  vol_loss_TLU=[.023, .023, .023, .023, .0285, .032; .0844, .0842, .0845, .084, .1125, .108; .1079, .108, .11, .108, .1605, .18] * 1e-3 m^3/s  mech_loss_TLU=[.002, .002, .002, .002, .002, .002; .0607, .0556, .0556, .0556, .0556, .0505; .1937, .1937, .1833, .1833, .1729, .1626] N*m  vol_eff_min=1e-3  vol_eff_max=1  mech_eff_min=1e-3  mech_eff_max=1  pressure_threshold=1e-3 MPa  omega_threshold=10 rad/s  supplied_range_check=simscape.enum.assert.action.none  pump_mode_check=simscape.enum.assert.action.none  pressure_check=simscape.enum.assert.action.none  p_min_valid=0.101325 MPa
  Reservoir (IL) : fl_lib/Isothermal Liquid/Elements/Reservoir (IL)  pressure_input=false  pressure_spec=foundation.enum.pressure_spec.atmospheric  reservoir_pressure=0.101325 MPa
  Outlet : PMIOPort  Side=Right
  C : PMIOPort  Port=2  Side=Left
  connections:
  C/RConn1 -- Pump/RConn1
  Pump/RConn2 -- Mechanical Rotational Reference/LConn1
  Pump/RConn3 -- Pressure Relief Valve/RConn1 -- Reservoir (IL)/LConn1
  Pressure Relief Valve/LConn1 -- Pump/LConn1 -- Outlet/RConn1

== system cvt_powertrain_lib/CVT Power Split Hydromechanical/Hydrostatic/Motor Leakage ==
  Case Drain : fl_lib/Isothermal Liquid/Elements/Reservoir (IL)  pressure_input=false  pressure_spec=foundation.enum.pressure_spec.atmospheric  reservoir_pressure=0.101325 MPa
  Leakage A : fl_lib/Isothermal Liquid/Elements/Laminar Leakage (IL)  cross_section_geometry=foundation.enum.cross_section_geometry.custom  diameter=1e-3 m  inner_diameter=5e-4 m  outer_diameter=1e-3 m  width=1e-3 m  height=0.1 m  major_axis=1e-3 m  minor_axis=5e-4 m  side_length=1e-3 m  length=5 m  resistance=1e7 s*MPa/m^3
  Leakage B : fl_lib/Isothermal Liquid/Elements/Laminar Leakage (IL)  cross_section_geometry=foundation.enum.cross_section_geometry.custom  diameter=1e-3 m  inner_diameter=5e-4 m  outer_diameter=1e-3 m  width=1e-3 m  height=0.1 m  major_axis=1e-3 m  minor_axis=5e-4 m  side_length=1e-3 m  length=5 m  resistance=1e7 s*MPa/m^3
  A : PMIOPort  Side=Left
  B : PMIOPort  Port=2  Side=Left
  connections:
  Leakage A/LConn1 -- A/RConn1
  Leakage B/RConn1 -- Case Drain/LConn1 -- Leakage A/RConn1
  Leakage B/LConn1 -- B/RConn1

== system cvt_powertrain_lib/CVT Power Split Hydromechanical/Hydrostatic/Pump Leakage ==
  Case Drain : fl_lib/Isothermal Liquid/Elements/Reservoir (IL)  pressure_input=false  pressure_spec=foundation.enum.pressure_spec.atmospheric  reservoir_pressure=0.101325 MPa
  Leakage A : fl_lib/Isothermal Liquid/Elements/Laminar Leakage (IL)  cross_section_geometry=foundation.enum.cross_section_geometry.custom  diameter=1e-3 m  inner_diameter=5e-4 m  outer_diameter=1e-3 m  width=1e-3 m  height=0.1 m  major_axis=1e-3 m  minor_axis=5e-4 m  side_length=1e-3 m  length=5 m  resistance=1e7 s*MPa/m^3
  Leakage B : fl_lib/Isothermal Liquid/Elements/Laminar Leakage (IL)  cross_section_geometry=foundation.enum.cross_section_geometry.custom  diameter=1e-3 m  inner_diameter=5e-4 m  outer_diameter=1e-3 m  width=1e-3 m  height=0.1 m  major_axis=1e-3 m  minor_axis=5e-4 m  side_length=1e-3 m  length=5 m  resistance=1e7 s*MPa/m^3
  B : PMIOPort  Side=Left
  A : PMIOPort  Port=2  Side=Left
  connections:
  Leakage A/LConn1 -- A/RConn1
  Leakage B/RConn1 -- Leakage A/RConn1 -- Case Drain/LConn1
  Leakage B/LConn1 -- B/RConn1

== system cvt_powertrain_lib/Controller/CVT Ratio Ctrl/Range Calculation ==
  Ratio (-) : Inport
  Check Range 0 or higher : Switch  Threshold=XY_I(1,2)  SaturateOnIntegerOverflow=off  InputSameDT=off
  Check Range 2 or higher : Switch  Threshold=XY_I(2,2)  SaturateOnIntegerOverflow=off  InputSameDT=off
  Check Range 3 or higher : Switch  Threshold=XY_I(3,2)  SaturateOnIntegerOverflow=off  InputSameDT=off
  Check Range 4 : Switch  Threshold=XY_I(4,2)  SaturateOnIntegerOverflow=off  InputSameDT=off
  Constant1 : Constant  Value=2  SampleTime=HMPST.Simu.TimeStep
  Constant2 : Constant  SampleTime=HMPST.Simu.TimeStep
  Constant3 : Constant  Value=-1  SampleTime=HMPST.Simu.TimeStep
  Constant4 : Constant  Value=3  SampleTime=HMPST.Simu.TimeStep
  Constant5 : Constant  Value=4  SampleTime=HMPST.Simu.TimeStep
  Range (-) : Outport
  wires:
  Check Range 2 or higher/1 -> Check Range 0 or higher/1
  Constant2/1 -> Check Range 2 or higher/3
  Constant3/1 -> Check Range 0 or higher/3
  Check Range 0 or higher/1 -> Range (-)/1  "Range"
  Check Range 3 or higher/1 -> Check Range 2 or higher/1
  Constant1/1 -> Check Range 3 or higher/3
  Check Range 4/1 -> Check Range 3 or higher/1
  Constant4/1 -> Check Range 4/3
  Constant5/1 -> Check Range 4/1
  Ratio (-)/1 -> Check Range 2 or higher/2, Check Range 3 or higher/2, Check Range 4/2, Check Range 0 or higher/2

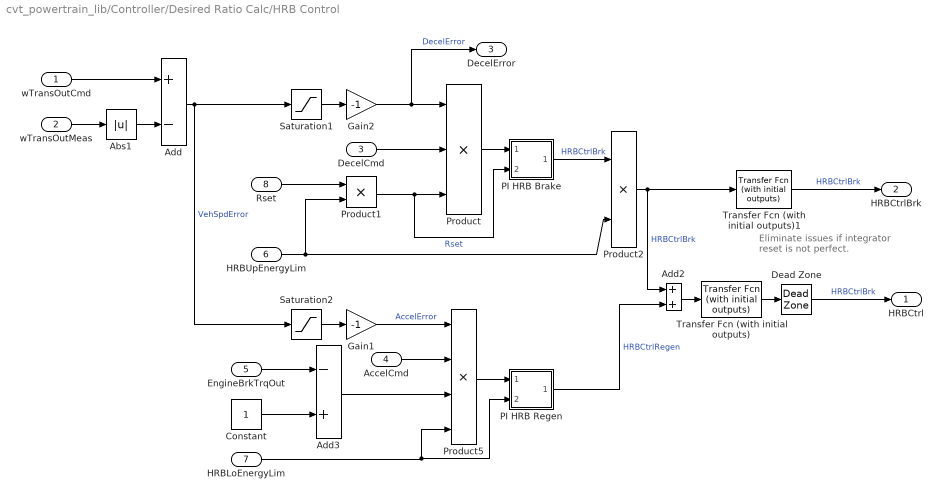
== system cvt_powertrain_lib/Controller/Desired Ratio Calc/HRB Control ==
  note: Eliminate issues if integrator reset is not perfect.
  wTransOutCmd : Inport
  wTransOutMeas : Inport  Port=2
  DecelCmd : Inport  Port=3
  AccelCmd : Inport  Port=4
  EngineBrkTrqOut : Inport  Port=5
  HRBUpEnergyLim : Inport  Port=6
  HRBLoEnergyLim : Inport  Port=7
  Rset : Inport  Port=8
  Abs1 : Abs  ZeroCross=off  SaturateOnIntegerOverflow=off
  Add : Sum  Inputs=+-
  Add2 : Sum
  Add3 : Sum  Inputs=-+
  Constant : Constant
  Dead Zone : DeadZone  LowerValue=-3e-3  UpperValue=3e-3
  Gain1 : Gain  Gain=-1
  Gain2 : Gain  Gain=-1
  PI HRB Brake : Subsystem
  PI HRB Regen : Subsystem
  Product : Product  Inputs=3
  Product1 : Product
  Product2 : Product
  Product5 : Product  Inputs=4
  Saturation1 : Saturate  UpperLimit=0  LowerLimit=-inf  ZeroCross=off
  Saturation2 : Saturate  UpperLimit=inf  LowerLimit=0  ZeroCross=off
  Transfer Fcn (with initial outputs) : simulink_extras/Additional Linear/Transfer Fcn (with initial outputs)  N=[0.01]  D=[0.05 1]  Y0=0  U0=0
  Transfer Fcn (with initial outputs)1 : simulink_extras/Additional Linear/Transfer Fcn (with initial outputs)  N=[0.01]  D=[0.05 1]  Y0=0  U0=0
  HRBCtrl : Outport
  HRBCtrlBrk : Outport  Port=2
  DecelError : Outport  Port=3
  wires:
  Transfer Fcn (with initial outputs)/1 -> Dead Zone/1
  Product/1 -> PI HRB Brake/1(error)
  Product5/1 -> PI HRB Regen/1(error)
  Gain1/1 -> Product5/1  "AccelError"
  Transfer Fcn (with initial outputs)1/1 -> HRBCtrlBrk/1  "HRBCtrlBrk"
  Rset/1 -> Product1/1
  EngineBrkTrqOut/1 -> Add3/1
  wTransOutCmd/1 -> Add/1
  PI HRB Brake/1(ctrl) -> Product2/1  "HRBCtrlBrk"
  wTransOutMeas/1 -> Abs1/1
  Gain2/1 -> Product/1, DecelError/1  "DecelError"
  AccelCmd/1 -> Product5/2
  Saturation1/1 -> Gain2/1
  Saturation2/1 -> Gain1/1
  PI HRB Regen/1(ctrl) -> Add2/2  "HRBCtrlRegen"
  HRBUpEnergyLim/1 -> Product2/2, Product1/2
  Abs1/1 -> Add/2
  DecelCmd/1 -> Product/2
  Product2/1 -> Add2/1, Transfer Fcn (with initial outputs)1/1  "HRBCtrlBrk"
  Add/1 -> Saturation1/1, Saturation2/1  "VehSpdError"
  Dead Zone/1 -> HRBCtrl/1  "HRBCtrlBrk"
  Constant/1 -> Add3/2
  Product1/1 -> Product/3, PI HRB Brake/2(Rset)  "Rset"
  Add3/1 -> Product5/3
  HRBLoEnergyLim/1 -> Product5/4, PI HRB Regen/2(Rset)
  Add2/1 -> Transfer Fcn (with initial outputs)/1

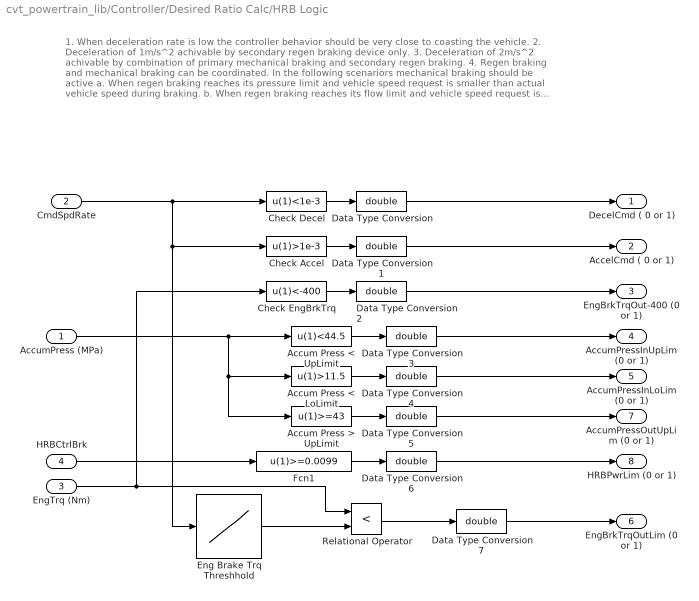
== system cvt_powertrain_lib/Controller/Desired Ratio Calc/HRB Logic ==
  note: 1. When deceleration rate is low the controller behavior should be very close to coasting the vehicle.
      | 2. Deceleration of 1m/s^2 achivable by secondary regen braking device only.
      | 3. Deceleration of 2m/s^2 achivable by combination of primary mechanical braking and secondary regen braking.
      | 4. Regen braking and mechanical braking can be coordinated. In the following scenariors mechanical braking should be active
      | a. When regen braking reaches its pressure limit and vehicle speed request is smaller than actual vehicle speed during braking.
      | b. When regen braking reaches its flow limit and vehicle speed request is smaller than actual vehicle speed during braking.
      | 5. Energy in the accumulator will be released when accelerating and the accumulator pressure is above minimum working pressure.
      | Energy release rate should not cause engine over speeding.
      | 6. If engine over speed limit is reached disengage master clutch/shut down the engine.
  AccumPress (MPa) : Inport
  CmdSpdRate : Inport  Port=2
  EngTrq (Nm) : Inport  Port=3
  HRBCtrlBrk : Inport  Port=4
  Accum Press < LoLimit : Fcn  Expr=u(1)>11.5
  Accum Press < UpLimit : Fcn  Expr=u(1)<44.5
  Accum Press > UpLimit : Fcn  Expr=u(1)>=43
  Check Accel : Fcn  Expr=u(1)>1e-3
  Check Decel : Fcn  Expr=u(1)<1e-3
  Check EngBrkTrq : Fcn  Expr=u(1)<-400
  Data Type Conversion{,1..7} (8 alike) : DataTypeConversion  OutDataTypeStr=double  SaturateOnIntegerOverflow=off  RndMeth=Floor
  Eng Brake Trq Threshhold : Lookup_n-D  NumberOfTableDimensions=1  BreakpointsForDimension1=[-3 -2 -1 -0.5 0 1]  Table=[-450 -450 -225 -113 0 0]*0.6  InternalRulePriority=Speed  RndMeth=Simplest
  Fcn1 : Fcn  Expr=u(1)>=0.0099
  Relational Operator : RelationalOperator  Operator=<  OutDataTypeStr=boolean  ZeroCross=off  InputSameDT=off
  DecelCmd ( 0 or 1) : Outport
  AccelCmd ( 0 or 1) : Outport  Port=2
  EngBrkTrqOut-400 (0 or 1) : Outport  Port=3
  AccumPressInUpLim (0 or 1) : Outport  Port=4
  AccumPressInLoLim (0 or 1) : Outport  Port=5
  EngBrkTrqOutLim (0 or 1) : Outport  Port=6
  AccumPressOutUpLim (0 or 1) : Outport  Port=7
  HRBPwrLim (0 or 1) : Outport  Port=8
  wires:
  Check Decel/1 -> Data Type Conversion/1
  Data Type Conversion/1 -> DecelCmd ( 0 or 1)/1
  EngTrq (Nm)/1 -> Relational Operator/1, Check EngBrkTrq/1
  CmdSpdRate/1 -> Check Decel/1, Eng Brake Trq Threshhold/1, Check Accel/1
  Eng Brake Trq Threshhold/1 -> Relational Operator/2
  AccumPress (MPa)/1 -> Accum Press < LoLimit/1, Accum Press > UpLimit/1, Accum Press < UpLimit/1
  Accum Press < UpLimit/1 -> Data Type Conversion3/1
  Relational Operator/1 -> Data Type Conversion7/1
  Accum Press > UpLimit/1 -> Data Type Conversion5/1
  HRBCtrlBrk/1 -> Fcn1/1
  Fcn1/1 -> Data Type Conversion6/1
  Accum Press < LoLimit/1 -> Data Type Conversion4/1
  Check Accel/1 -> Data Type Conversion1/1
  Check EngBrkTrq/1 -> Data Type Conversion2/1
  Data Type Conversion1/1 -> AccelCmd ( 0 or 1)/1
  Data Type Conversion2/1 -> EngBrkTrqOut-400 (0 or 1)/1
  Data Type Conversion3/1 -> AccumPressInUpLim (0 or 1)/1
  Data Type Conversion4/1 -> AccumPressInLoLim (0 or 1)/1
  Data Type Conversion5/1 -> AccumPressOutUpLim (0 or 1)/1
  Data Type Conversion6/1 -> HRBPwrLim (0 or 1)/1
  Data Type Conversion7/1 -> EngBrkTrqOutLim (0 or 1)/1
